simulink model "sampleModel1834"  (R2023a)
settings: Solver=VariableStepAuto  StartTime=0.0  StopTime=10.0  RelTol=1e-3
libraries: hdlsllib x4, simulink x4
settings Model: Creator=user1  LastModifiedBy=user1

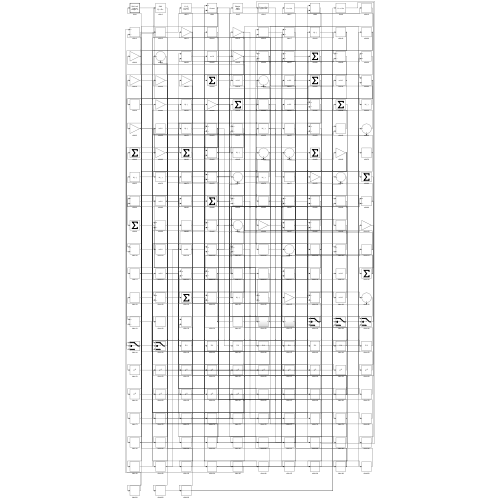
[thumbnail: Simulink's stored preview of the top-level diagram]
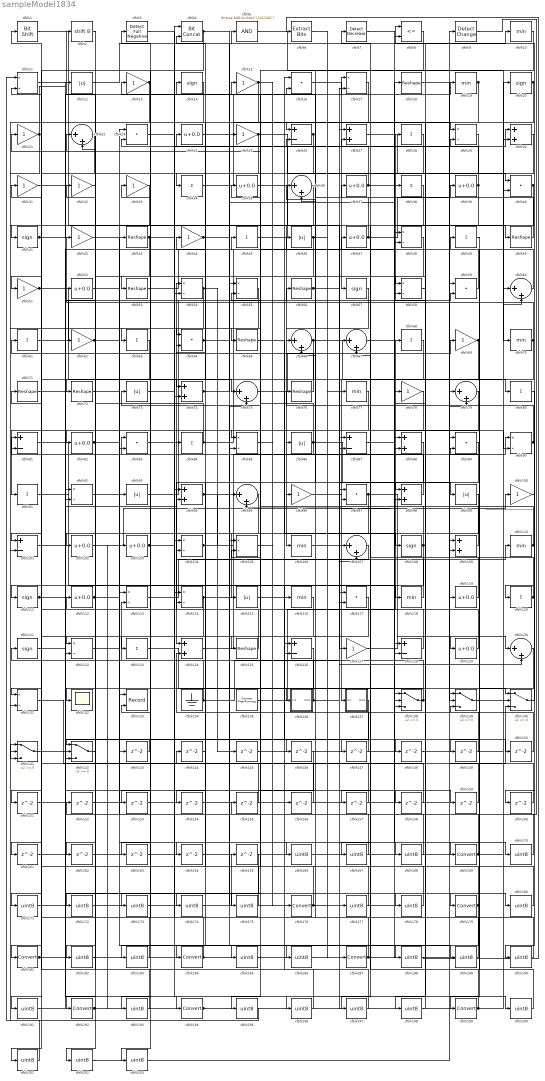
== system sampleModel1834 ==
  cfblk1 : hdlsllib/Logic and Bit Operations/Bit Shift  mode=Shift Left Logical  N=0
  cfblk{10,19,70,77,106,110,116,118} (8 alike) : MinMax
  cfblk{13,15,21,25,31..33,42,44,51,62,69,78,96,100,127} (16 alike) : Gain
  cfblk{26,81,87,101,126,128} (6 alike) : Sum  Inputs=+-
  cfblk{24,35,37,39,47,52,82,102..103,112,119,129} (12 alike) : Bias  Bias=0.0  SaturateOnIntegerOverflow=off
  cfblk{11,17,29,48,54..55,58,85,90,92,104..105,113..114,122,131} (16 alike) : Product  Inputs=*/  RndMeth=Zero  SaturateOnIntegerOverflow=on
  cfblk{22,36,60,66..67,75,79,95,107,130} (10 alike) : Sum  Inputs=|++
  cfblk{14,20,41,57,108,111,121} (7 alike) : Signum
  cfblk{27,30,74,88,94,98,109,124} (8 alike) : Sum
  cfblk{12,46,73,86,93,99,115} (7 alike) : Abs  SaturateOnIntegerOverflow=off
  cfblk{16,23,40,59,64,83,89,97,117} (9 alike) : DotProduct  OutDataTypeStr=Inherit: Inherit via internal rule
  cfblk{28,34,38,45,49,61,63,68,80,84,91,120,123} (13 alike) : Sum  Inputs=+
  cfblk{18,43,50,53,56,65,71..72,76,125} (10 alike) : Reshape
  cfblk132 : Scope
  cfblk133 : Record  FileSettingsInternal="{\"entries\":[{\"content\":{\"excelSettings\":{\"content\":{},\"type\":\"Streamout.ExcelSettings\"}},\"type\":\"Streamout.FileSettingStorage\",\"uuid\":\"\"}],\"packageUris\":[\"http:\\/\\/schema.mathworks.com\\/mf0\\/streamout_blocks\\/R2020a\"],\"version\":\"1.0\"}"  Layout=[1 1]  SignalsInternal="{\"entries\":[{\"content\":{\"signals\":[{\"content\":{\"blockPath\":[],\"dimensions\":[1],\"domain\":\"\",\"lineColor\":\"#a2142f\",\"plots\":[1],\"port\":1,\"signalID\":4464,\"signalName\":\"XY Graph:1\"},\"type\":\"RecordBlkView.Signal\",\"uuid\":\"\"},{\"content\":{\"blockPath\":[],\"dimensions\":[1],\"domain\":\"\",\"lineColor\":\"#139fff\",\"plots\":[1],\"port\":2,\"signalID\":4467,\"signalName\":\"XY Graph:2\"},\"type\":\"RecordBlkView.Signal\",\"uuid\":\"\"}]},\"type\":\"RecordBlkView.InputSignals\",\"uuid\":\"\"}],\"packageUris\":[\"http:\\/\\/schema.mathworks.com\\/mf0\\/streamout_blocks\\/R2020a\"],\"version\":\"1.0\"}"  VisualizationBindings="{\"xyplotplugin\":{\"info\":[{\"series\":[{\"bindingParametersList\":[{\"parameter\":\"X-Axis\",\"signalID\":4464,\"signalName\":\"XY Graph:1\"},{\"parameter\":\"Y-Axis\",\"signalID\":4467,\"signalName\":\"XY Graph:2\"}],\"seriesID\":65485}],\"subplotID\":1}]}}"  CompatibilityTag=XY  st=-1
  cfblk134 : Ground
  cfblk135 : hdlsllib/Sources/Counter Free-Running  NumBits=16  tsamp=-1
  cfblk136 : Subsystem
      settings: LibrarySourceBlock=|
      | hdlsllib/Ports &
      | Subsystems/Subsystem
  cfblk137 : Subsystem
      settings: LibrarySourceBlock=|
      | hdlsllib/Ports &
      | Subsystems/Subsystem
  cfblk{138..142} (5 alike) : Switch  SaturateOnIntegerOverflow=off  InputSameDT=off
  cfblk{143..165} (23 alike) : Delay  SampleTime=1
  cfblk{166..168,170..175,177..178,180,182..183,185..186,188..191,193,195..198,200..203} (29 alike) : DataTypeConversion  OutDataTypeStr=uint8  SaturateOnIntegerOverflow=off  RndMeth=Floor
  cfblk{169,176,179,181,184,187,192,194,199} (9 alike) : DataTypeConversion  SaturateOnIntegerOverflow=off  RndMeth=Floor
  cfblk2 : ArithShift  BitShiftNumber=8
  cfblk3 : hdlsllib/Logic and Bit Operations/Detect Fall Negative  vinit=0  OutDataTypeStr=boolean
  cfblk4 : hdlsllib/Logic and Bit Operations/Bit Concat  numInputs=2
  cfblk5 : simulink/Logic and Bit Operations/Bitwise Operator  logicop=AND  UseBitMask=on  BitMask=bin2dec('11011001')  BitMaskRealWorld=Stored Integer
      settings: LibrarySourceBlock=|
      | hdlsllib/Logic and Bit
      | Operations/Bitwise
      | Operator
  cfblk6 : simulink/Logic and Bit Operations/Extract Bits  bitsToExtract=Upper half  numBits=8  bitIdxRange=[0 7]  outScalingMode=Preserve fixed-point scaling
      settings: LibrarySourceBlock=|
      | hdlsllib/Logic and Bit
      | Operations/Extract Bits
  cfblk7 : simulink/Logic and Bit Operations/Detect Decrease  vinit=0.0  OutDataTypeStr=boolean
      settings: LibrarySourceBlock=|
      | hdlsllib/Logic and Bit
      | Operations/Detect
      | Decrease
  cfblk8 : RelationalOperator  Operator=<=  OutDataTypeStr=boolean  InputSameDT=off
  cfblk9 : simulink/Logic and Bit Operations/Detect Change  vinit=0  OutDataTypeStr=boolean
      settings: LibrarySourceBlock=|
      | hdlsllib/Logic and Bit
      | Operations/Detect
      | Change
  wires:
  cfblk129/1 -> cfblk112/1
  cfblk85/1 -> cfblk116/1
  cfblk34/1 -> cfblk17/1
  cfblk57/1 -> cfblk106/1
  cfblk121/1 -> cfblk179/1
  cfblk36/1 -> cfblk41/1
  cfblk47/1 -> cfblk39/1, cfblk16/2
  cfblk123/1 -> cfblk140/1
  cfblk46/1 -> cfblk53/1, cfblk177/1
  cfblk53/1 -> cfblk45/1
  cfblk70/1 -> cfblk42/1, cfblk167/1
  cfblk1/1 -> cfblk86/1
  cfblk16/1 -> cfblk57/1
  cfblk4/1 -> cfblk63/1, cfblk118/1, cfblk131/1
  cfblk15/1 -> cfblk64/1, cfblk156/1
  cfblk109/1 -> cfblk13/1
  cfblk135/1 -> cfblk68/1
  cfblk138/1 -> cfblk113/2, cfblk132/1
  cfblk99/1 -> cfblk122/1
  cfblk128/1 -> cfblk54/1
  cfblk50/1 -> cfblk15/1
  cfblk26/1 -> cfblk72/1, cfblk74/1
  cfblk22/1 -> cfblk181/1
  cfblk49/1 -> cfblk199/1
  cfblk84/1 -> cfblk17/2, cfblk138/2, cfblk12/1
  cfblk118/1 -> cfblk7/1
  cfblk88/1 -> cfblk124/1
  cfblk140/1 -> cfblk8/1
  cfblk74/1 -> cfblk59/2, cfblk148/1, cfblk186/1
  cfblk75/1 -> cfblk69/1
  cfblk41/1 -> cfblk19/1, cfblk191/1
  cfblk17/1 -> cfblk26/1
  cfblk69/1 -> cfblk137/1(In1), cfblk138/3, cfblk175/1
  cfblk39/1 -> cfblk66/1, cfblk3/1
  cfblk95/1 -> cfblk122/2
  cfblk102/1 -> cfblk100/1
  cfblk77/1 -> cfblk91/1
  cfblk14/1 -> cfblk51/1
  cfblk104/1 -> cfblk90/1, cfblk95/1
  cfblk125/1 -> cfblk71/1
  cfblk10/1 -> cfblk96/1
  cfblk6/1 -> cfblk187/1
  cfblk21/1 -> cfblk2/1, cfblk101/2
  cfblk27/1 -> cfblk40/1
  cfblk51/1 -> cfblk75/1, cfblk173/1
  cfblk137/1(Out1) -> cfblk142/1
  cfblk8/1 -> cfblk85/1
  cfblk124/1 -> cfblk40/2
  cfblk82/1 -> cfblk43/1, cfblk178/1
  cfblk76/1 -> cfblk61/1
  cfblk131/1 -> cfblk140/3
  cfblk113/1 -> cfblk110/1
  cfblk91/1 -> cfblk126/1
  cfblk37/1 -> cfblk88/1, cfblk26/2
  cfblk108/1 -> cfblk73/1, cfblk58/2, cfblk171/1
  cfblk67/1 -> cfblk90/2
  cfblk98/1 -> cfblk14/1
  cfblk97/1 -> cfblk130/1, cfblk115/1
  cfblk65/1 -> cfblk108/1
  cfblk127/1 -> cfblk129/1
  cfblk60/1 -> cfblk35/1
  cfblk45/1 -> cfblk30/1
  cfblk44/1 -> cfblk55/1, cfblk136/1(In1)
  cfblk93/1 -> cfblk28/1
  cfblk71/1 -> cfblk56/1
  cfblk114/1 -> cfblk9/1, cfblk153/1
  cfblk81/1 -> cfblk126/2
  cfblk110/1 -> cfblk46/1, cfblk95/2
  cfblk35/1 -> cfblk107/1
  cfblk54/1 -> cfblk102/1, cfblk131/2, cfblk145/1
  cfblk66/1 -> cfblk80/1, cfblk161/1
  cfblk19/1 -> cfblk58/1, cfblk125/1
  cfblk120/1 -> cfblk37/1, cfblk67/2
  cfblk25/1 -> cfblk34/1, cfblk89/1, cfblk162/1
  cfblk90/1 -> cfblk76/1, cfblk190/1
  cfblk87/1 -> cfblk169/1
  cfblk32/1 -> cfblk192/1
  cfblk7/1 -> cfblk50/1
  cfblk112/1 -> cfblk133/1, cfblk170/1
  cfblk42/1 -> cfblk93/1
  cfblk68/1 -> cfblk123/1
  cfblk30/1 -> cfblk128/2
  cfblk59/1 -> cfblk36/1
  cfblk43/1 -> cfblk84/1, cfblk83/2
  cfblk105/1 -> cfblk176/1
  cfblk96/1 -> cfblk97/2
  cfblk100/1 -> cfblk120/1
  cfblk18/1 -> cfblk109/1
  cfblk28/1 -> cfblk65/1
  cfblk64/1 -> cfblk10/1, cfblk38/1
  cfblk12/1 -> cfblk5/1
  cfblk63/1 -> cfblk111/1
  cfblk107/1 -> cfblk104/2
  cfblk117/1 -> cfblk184/1
  cfblk5/1 -> cfblk70/1
  cfblk103/1 -> cfblk29/2, cfblk163/1
  cfblk20/1 -> cfblk139/2, cfblk193/1
  cfblk106/1 -> cfblk127/1
  cfblk62/1 -> cfblk164/1, cfblk168/1
  cfblk86/1 -> cfblk98/1, cfblk21/1, cfblk81/2
  cfblk134/1 -> cfblk27/1, cfblk81/1
  cfblk3/1 -> cfblk94/1
  cfblk2/1 -> cfblk82/1
  cfblk11/1 -> cfblk194/1
  cfblk136/1(Out1) -> cfblk33/1, cfblk130/2
  cfblk111/1 -> cfblk94/2, cfblk48/2
  cfblk142/1 -> cfblk52/1
  cfblk56/1 -> cfblk99/1, cfblk77/1
  cfblk24/1 -> cfblk29/1
  cfblk13/1 -> cfblk141/2, cfblk142/3
  cfblk40/1 -> cfblk101/1, cfblk141/3
  cfblk61/1 -> cfblk25/1
  cfblk139/1 -> cfblk60/2
  cfblk94/1 -> cfblk24/1, cfblk18/1
  cfblk119/1 -> cfblk83/1
  cfblk52/1 -> cfblk143/1
  cfblk143/1 -> cfblk142/2
  cfblk145/1 -> cfblk138/1
  cfblk141/1 -> cfblk146/1
  cfblk72/1 -> cfblk147/1
  cfblk147/1 -> cfblk55/2
  cfblk148/1 -> cfblk60/1
  cfblk130/1 -> cfblk149/1
  cfblk149/1 -> cfblk124/2
  cfblk115/1 -> cfblk150/1
  cfblk150/1 -> cfblk36/2
  cfblk116/1 -> cfblk151/1
  cfblk151/1 -> cfblk85/2
  cfblk9/1 -> cfblk152/1
  cfblk152/1 -> cfblk128/1
  cfblk153/1 -> cfblk107/2
  cfblk89/1 -> cfblk154/1
  cfblk154/1 -> cfblk139/1
  cfblk155/1 -> cfblk4/2
  cfblk156/1 -> cfblk1/1
  cfblk38/1 -> cfblk157/1
  cfblk157/1 -> cfblk113/1
  cfblk122/1 -> cfblk158/1
  cfblk158/1 -> cfblk104/1
  cfblk31/1 -> cfblk159/1
  cfblk159/1 -> cfblk59/1
  cfblk80/1 -> cfblk160/1
  cfblk160/1 -> cfblk139/3
  cfblk161/1 -> cfblk74/2
  cfblk162/1 -> cfblk54/2
  cfblk163/1 -> cfblk30/2
  cfblk164/1 -> cfblk88/2
  cfblk23/1 -> cfblk166/1
  cfblk166/1 -> cfblk140/2
  cfblk167/1 -> cfblk23/1
  cfblk168/1 -> cfblk23/2
  cfblk169/1 -> cfblk155/1, cfblk89/2, cfblk114/2, cfblk8/2
  cfblk170/1 -> cfblk87/1
  cfblk171/1 -> cfblk87/2
  cfblk165/1 -> cfblk172/1
  cfblk172/1 -> cfblk98/2
  cfblk173/1 -> cfblk165/1
  cfblk144/1 -> cfblk174/1
  cfblk174/1 -> cfblk75/2
  cfblk175/1 -> cfblk144/1
  cfblk176/1 -> cfblk64/2, cfblk114/1
  cfblk177/1 -> cfblk105/1
  cfblk178/1 -> cfblk105/2
  cfblk179/1 -> cfblk44/1, cfblk203/1
  cfblk101/1 -> cfblk180/1
  cfblk180/1 -> cfblk121/1
  cfblk181/1 -> cfblk62/1, cfblk119/1
  cfblk33/1 -> cfblk182/1
  cfblk182/1 -> cfblk22/1
  cfblk55/1 -> cfblk183/1
  cfblk183/1 -> cfblk22/2
  cfblk184/1 -> cfblk48/1, cfblk133/2, cfblk31/1
  cfblk126/1 -> cfblk185/1
  cfblk185/1 -> cfblk117/1
  cfblk186/1 -> cfblk117/2
  cfblk187/1 -> cfblk4/1, cfblk97/1
  cfblk58/1 -> cfblk188/1
  cfblk188/1 -> cfblk6/1
  cfblk92/1 -> cfblk189/1
  cfblk189/1 -> cfblk66/2
  cfblk190/1 -> cfblk92/1
  cfblk191/1 -> cfblk92/2
  cfblk192/1 -> cfblk67/1, cfblk103/1
  cfblk193/1 -> cfblk32/1
  cfblk194/1 -> cfblk20/1, cfblk109/2
  cfblk146/1 -> cfblk195/1
  cfblk195/1 -> cfblk11/1
  cfblk83/1 -> cfblk196/1
  cfblk196/1 -> cfblk11/2
  cfblk78/1 -> cfblk197/1
  cfblk197/1 -> cfblk16/1
  cfblk29/1 -> cfblk198/1
  cfblk198/1 -> cfblk78/1
  cfblk199/1 -> cfblk27/2, cfblk47/1
  cfblk73/1 -> cfblk200/1
  cfblk200/1 -> cfblk49/1
  cfblk79/1 -> cfblk201/1
  cfblk201/1 -> cfblk141/1
  cfblk48/1 -> cfblk202/1
  cfblk202/1 -> cfblk79/1
  cfblk203/1 -> cfblk79/2

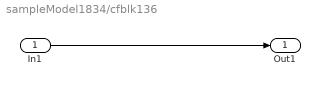
== system sampleModel1834/cfblk136 ==
  In1 : Inport
  Out1 : Outport
  wires:
  In1/1 -> Out1/1

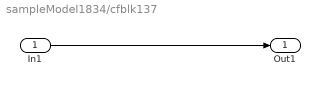
== system sampleModel1834/cfblk137 ==
  In1 : Inport
  Out1 : Outport
  wires:
  In1/1 -> Out1/1
